simulink model "rtwdemo_rtwintro"  (Simulink 7.6)
settings: Solver=FixedStepDiscrete  StartTime=0.0  StopTime=48  FixedStep=1  RelTol=1e-3  SampleTimeConstraint=STIndependent
PostLoadFcn:
  | INC=uint8(1);LIMIT=uint8(16);RESET=uint8(0);K=int32(2);
Description:
  | Generating Code Using the Real-Time Workshop Product
settings Model: Creator=The MathWorks Inc.  ParamWorkspaceSource=ReferencedWorkspace  CovMetricSettings=d  ExtModeTrigMode=oneshot  ExtModeArmWhenConnect=off  ExtModeAutoUpdateStatusClock=off
settings MATStruct: SampleTime=1  Offset=0  Priority=[41.0]
settings DataIOCC: LimitDataPoints=off  SaveFormat=StructureWithTime  SaveOutput=off  SaveTime=off  SignalLoggingName=sigsOut
settings OptimizationCC: InlineParams=on  InlineInvariantSignals=on  StateBitsets=on  DataBitsets=on  UseTempVars=on  EfficientFloat2IntCast=on  EfficientMapNaN2IntZero=off  BufferReusableBoundary=off
settings DebuggingCC: UnderspecifiedInitializationDetection=Simplified  MergeDetectMultiDrivingBlocksExec=error  CheckExecutionContextPreStartOutputMsg=on  CheckExecutionContextRuntimeOutputMsg=on  SolverPrmCheckMsg=none  IntegerOverflowMsg=none  UniqueDataStoreMsg=error  StrictBusMsg=ErrorOnBusTreatedAsVector
settings HardwareCC: ProdIntDivRoundTo=Zero  ProdEndianess=LittleEndian  ProdHWDeviceType=Generic->32-bit Embedded Processor  TargetHWDeviceType=Generic->32-bit Embedded Processor
settings ModelReferenceCC: UpdateModelReferenceTargets=IfOutOfDate
settings RTWCC: TLCOptions=-p0  GenerateReport=on  RTWVerbose=off  ProcessScript=grt_make_rtw_hook  LaunchReport=on
settings CodeAppCC: ForceParamTrailComments=on

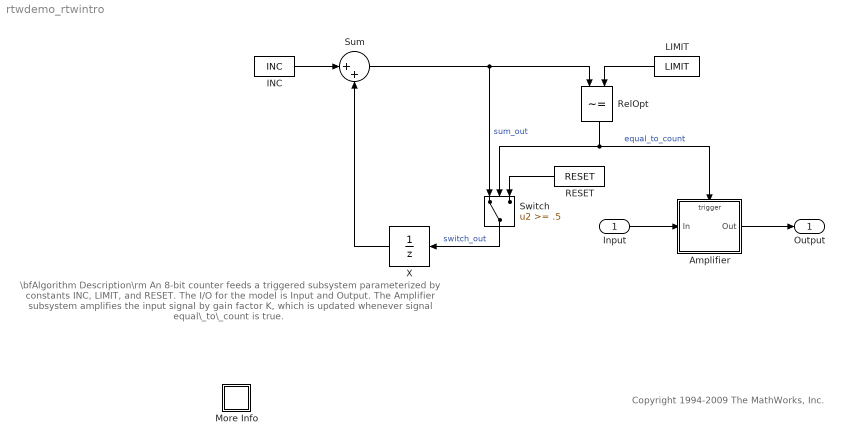
== system rtwdemo_rtwintro ==
  note: \bfAlgorithm Description\rm
      | An 8-bit counter feeds a triggered subsystem parameterized by constants INC, LIMIT, and RESET.
      | The I/O for the model is Input and Output. The Amplifier subsystem amplifies the input signal by
      | gain factor K, which is updated whenever signal equal\_to\_count  is true.
  note: Copyright 1994-2009 The MathWorks, Inc.
  Input : Inport  OutDataTypeStr=int32  PortDimensions=1
  Amplifier : Subsystem  TreatAsAtomicUnit=on
  INC : Constant  Value=INC
  LIMIT : Constant  Value=LIMIT
  More Info : Subsystem
      settings: OpenFcn=showdemo('rtwdemo_usingrtw')
      mask Display: disp('?')
  RESET : Constant  Value=RESET
  RelOpt : RelationalOperator  Operator=~=  InputSameDT=on
  Sum : Sum  Inputs=|++  InputSameDT=on  OutDataTypeStr=Inherit: Same as first input
  Switch : Switch  Threshold=.5  InputSameDT=on
  X : UnitDelay  SampleTime=-1  StateIdentifier=X
  Output : Outport
  wires:
  INC/1 -> Sum/1
  X/1 -> Sum/2
  Switch/1 -> X/1  "switch_out"
  Sum/1 -> Switch/1, RelOpt/1  "sum_out"
  LIMIT/1 -> RelOpt/2
  Input/1 -> Amplifier/1(In)
  RESET/1 -> Switch/3
  RelOpt/1 -> Switch/2, Amplifier/Trigger  "equal_to_count"
  Amplifier/1(Out) -> Output/1

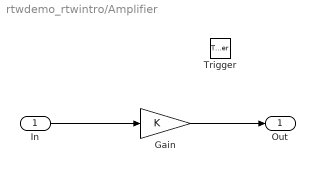
== system rtwdemo_rtwintro/Amplifier ==
  In : Inport
  Trigger : TriggerPort
  Gain : Gain  Gain=K  OutDataTypeStr=Inherit: Same as input  ParamDataTypeStr=Inherit: Same as input
  Out : Outport  InitialOutput=0
  wires:
  In/1 -> Gain/1
  Gain/1 -> Out/1

== system rtwdemo_rtwintro/More Info ==
